simulink subsystem "Open_Differential_with_loss"  (R2022b)
settings: Solver=VariableStepAuto  StartTime=0.0  StopTime=10.0  RelTol=1e-3
undefined symbols (not defined in the file): Diff_EffMap, Diff_Spd_BrkPts, Diff_Trq_BrkPts, PlntDiffrntlAxl1Damp, PlntDiffrntlCarrDamp, PlntDiffrntlEff, PlntDiffrntlPwrThresh
libraries: fl_lib x7, nesl_utility x7, sdl_lib x1
settings Model: Creator=Thomas  LastModifiedBy=Thomas

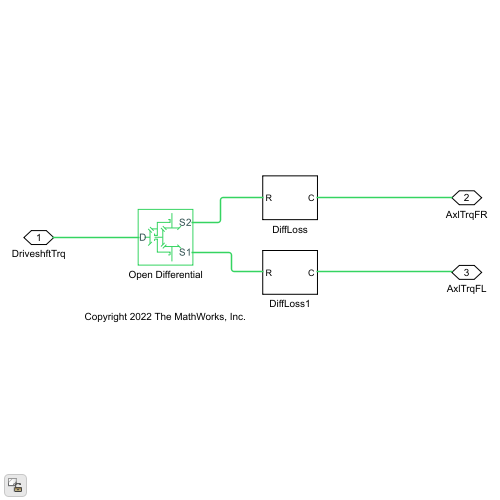
[thumbnail: Simulink's stored preview of the top-level diagram]
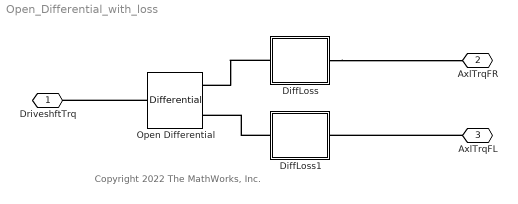
== system Open_Differential_with_loss ==
  note: Copyright 2022 The MathWorks, Inc.
  DiffLoss : Subsystem
  DiffLoss1 : Subsystem
  Open Differential : sdl_lib/Gears/Differential  driveshaft_location=sdl.enum.differential_orientation.right  cd_ratio=PlntDiffrntlRatio  friction_model=sdl.enum.gear_friction.constant  efficiency=[PlntDiffrntlEff PlntDiffrntlEff]  temperature_TLU=[280, 300, 320] K  efficiency_ss_TLU=[.95, .9, .85]  efficiency_cd_TLU=[.95, .9, .85]  pwr_thr=[PlntDiffrntlPwrThresh, PlntDiffrntlPwrThresh] W  mu_visc=[PlntDiffrntlCarrDamp PlntDiffrntlAxl1Damp] N*m*s/rad  model_inertia=simscape.enum.onoff.off  carrier_inertia=PlntDiffrntlCarrInertia kg*m^2  planet_inertia=PlntDiffrntlAxl1Inertia kg*m^2  thermal_mass=50 J/K  T_init=300 K
  DriveshftTrq : PMIOPort  Side=Left
  AxlTrqFR : PMIOPort  Port=2  Side=Right
  AxlTrqFL : PMIOPort  Port=3  Side=Right
  connections:
  AxlTrqFL/RConn1 -- DiffLoss1/RConn1
  DiffLoss/LConn1 -- Open Differential/RConn2
  Open Differential/LConn1 -- DriveshftTrq/RConn1
  DiffLoss1/LConn1 -- Open Differential/RConn1
  DiffLoss/RConn1 -- AxlTrqFR/RConn1

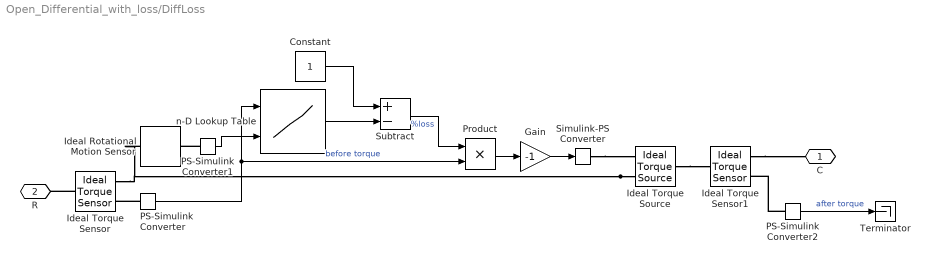
== system Open_Differential_with_loss/DiffLoss ==
  Constant : Constant
  Gain : Gain  Gain=-1
  Ideal Rotational Motion Sensor : fl_lib/Mechanical/Mechanical Sensors/Ideal Rotational Motion Sensor  reference=foundation.enum.MeasurementReference.absolute  acceleration_port=false  velocity_port=true  position_port=false  wrap_angle=false  offset=0 rad
      settings: InternalSimscapePortConfiguration="{\"Bottom\":[],\"Left\":[{\"id\":\"R\",\"label\":\"R\",\"type\":\"foundation.mechanical.rotational.rotational\"}],\"Right\":[{\"id\":\"W\",\"label\":\"W\",\"type\":\"output\"}],\"Top\":[]}"
  Ideal Torque Sensor : fl_lib/Mechanical/Mechanical Sensors/Ideal Torque Sensor
  Ideal Torque Sensor1 : fl_lib/Mechanical/Mechanical Sensors/Ideal Torque Sensor
  Ideal Torque Source : fl_lib/Mechanical/Mechanical Sources/Ideal Torque Source
  PS-Simulink Converter : nesl_utility/PS-Simulink Converter  PhysicalDomain=network_engine_domain  SubClassName=ps_output  LeftPortType=input  RightPortType=output  PseudoPeriodic=off  Frequencies=[]  VectorFormat=inherit  Unit=inherit  AffineConversion=off
  PS-Simulink Converter1 : nesl_utility/PS-Simulink Converter  PhysicalDomain=network_engine_domain  SubClassName=ps_output  LeftPortType=input  RightPortType=output  PseudoPeriodic=off  Frequencies=[]  VectorFormat=inherit  Unit=inherit  AffineConversion=off
  PS-Simulink Converter2 : nesl_utility/PS-Simulink Converter  PhysicalDomain=network_engine_domain  SubClassName=ps_output  LeftPortType=input  RightPortType=output  PseudoPeriodic=off  Frequencies=[]  VectorFormat=inherit  Unit=inherit  AffineConversion=off
  Product : Product
  Simulink-PS Converter : nesl_utility/Simulink-PS Converter  PhysicalDomain=network_engine_domain  SubClassName=ps_input  LeftPortType=input  RightPortType=output  PseudoPeriodic=off  Frequencies=[]  NoiseDistribution=none  NoiseParameters=[]  Unit=1  AffineConversion=off  FilteringAndDerivatives=provide  SimscapeFilterOrder=1  InputFilterTimeConstant=0.001  UdotUserProvided=0
  Subtract : Sum  Inputs=+-
  Terminator : Terminator
  n-D Lookup Table : Lookup_n-D  BreakpointsForDimension1=Diff_Trq_BrkPts  BreakpointsForDimension2=Diff_Spd_BrkPts  BreakpointsForDimension3=[5, 7]  Table=Diff_EffMap  InternalRulePriority=Speed  RndMeth=Simplest
      settings: InputPortMap=u0,u1
  C : PMIOPort  Side=Right
  R : PMIOPort  Port=2  Side=Left
  wires:
  PS-Simulink Converter2/1 -> Terminator/1  "after torque"
  PS-Simulink Converter1/1 -> n-D Lookup Table/2
  Gain/1 -> Simulink-PS Converter/1
  Product/1 -> Gain/1
  n-D Lookup Table/1 -> Subtract/2
  Subtract/1 -> Product/1  "%loss"
  Constant/1 -> Subtract/1
  PS-Simulink Converter/1 -> Product/2, n-D Lookup Table/1  "before torque"
  connections:
  Ideal Torque Sensor1/RConn1 -- C/RConn1
  Ideal Torque Source/LConn1 -- Ideal Torque Sensor1/LConn1
  PS-Simulink Converter2/LConn1 -- Ideal Torque Sensor1/RConn2
  Simulink-PS Converter/RConn1 -- Ideal Torque Source/RConn1
  PS-Simulink Converter1/LConn1 -- Ideal Rotational Motion Sensor/RConn1
  Ideal Torque Sensor/LConn1 -- R/RConn1
  Ideal Torque Source/RConn2 -- Ideal Rotational Motion Sensor/LConn1 -- Ideal Torque Sensor/RConn1
  PS-Simulink Converter/LConn1 -- Ideal Torque Sensor/RConn2

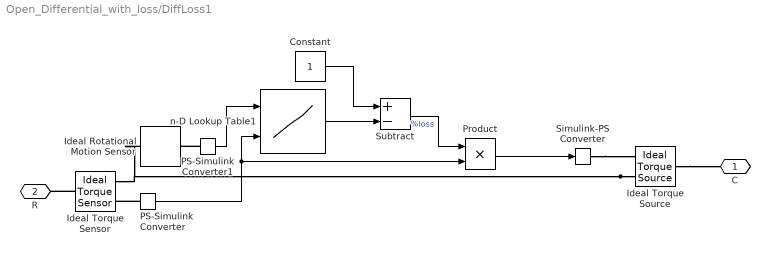
== system Open_Differential_with_loss/DiffLoss1 ==
  Constant : Constant
  Ideal Rotational Motion Sensor : fl_lib/Mechanical/Mechanical Sensors/Ideal Rotational Motion Sensor  reference=foundation.enum.MeasurementReference.absolute  acceleration_port=false  velocity_port=true  position_port=false  wrap_angle=false  offset=0 rad
      settings: InternalSimscapePortConfiguration="{\"Bottom\":[],\"Left\":[{\"id\":\"R\",\"label\":\"R\",\"type\":\"foundation.mechanical.rotational.rotational\"}],\"Right\":[{\"id\":\"W\",\"label\":\"W\",\"type\":\"output\"}],\"Top\":[]}"
  Ideal Torque Sensor : fl_lib/Mechanical/Mechanical Sensors/Ideal Torque Sensor
  Ideal Torque Source : fl_lib/Mechanical/Mechanical Sources/Ideal Torque Source
  PS-Simulink Converter : nesl_utility/PS-Simulink Converter  PhysicalDomain=network_engine_domain  SubClassName=ps_output  LeftPortType=input  RightPortType=output  PseudoPeriodic=off  Frequencies=[]  VectorFormat=inherit  Unit=inherit  AffineConversion=off
  PS-Simulink Converter1 : nesl_utility/PS-Simulink Converter  PhysicalDomain=network_engine_domain  SubClassName=ps_output  LeftPortType=input  RightPortType=output  PseudoPeriodic=off  Frequencies=[]  VectorFormat=inherit  Unit=inherit  AffineConversion=off
  Product : Product
  Simulink-PS Converter : nesl_utility/Simulink-PS Converter  PhysicalDomain=network_engine_domain  SubClassName=ps_input  LeftPortType=input  RightPortType=output  PseudoPeriodic=off  Frequencies=[]  NoiseDistribution=none  NoiseParameters=[]  Unit=1  AffineConversion=off  FilteringAndDerivatives=provide  SimscapeFilterOrder=1  InputFilterTimeConstant=0.001  UdotUserProvided=0
  Subtract : Sum  Inputs=+-
  n-D Lookup Table1 : Lookup_n-D  BreakpointsForDimension1=Diff_Trq_BrkPts  BreakpointsForDimension2=Diff_Spd_BrkPts  BreakpointsForDimension3=[5, 7]  Table=Diff_EffMap  InternalRulePriority=Speed  RndMeth=Simplest
      settings: InputPortMap=u0,u1
  C : PMIOPort  Side=Right
  R : PMIOPort  Port=2  Side=Left
  wires:
  Product/1 -> Simulink-PS Converter/1
  n-D Lookup Table1/1 -> Subtract/2
  Subtract/1 -> Product/1  "%loss"
  Constant/1 -> Subtract/1
  PS-Simulink Converter1/1 -> n-D Lookup Table1/1
  PS-Simulink Converter/1 -> Product/2, n-D Lookup Table1/2
  connections:
  Simulink-PS Converter/RConn1 -- Ideal Torque Source/RConn1
  Ideal Torque Source/LConn1 -- C/RConn1
  PS-Simulink Converter1/LConn1 -- Ideal Rotational Motion Sensor/RConn1
  Ideal Torque Sensor/LConn1 -- R/RConn1
  Ideal Torque Source/RConn2 -- Ideal Rotational Motion Sensor/LConn1 -- Ideal Torque Sensor/RConn1
  PS-Simulink Converter/LConn1 -- Ideal Torque Sensor/RConn2
